simulink model "dsp_blr_AveOnly"  (R2018a)
settings: Solver=VariableStepAuto  StartTime=0.0  StopTime=100e-6  RelTol=1e-3
libraries: xrbsSSR_Library x26, xbsIndex_r4 x16, dspsigattribs x1, hdlsllib x1, simulink x1
(part 2 of 2)

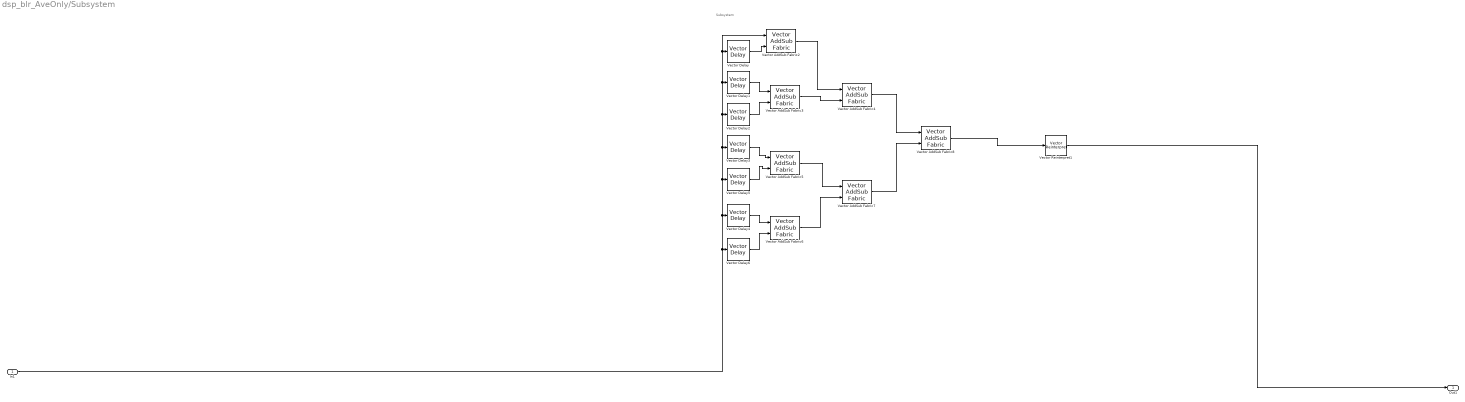
== system dsp_blr_AveOnly/Subsystem ==
  note: Subsystem
  In1 : Inport
  Vector AddSub Fabric{2..8} (7 alike) : xrbsSSR_Library/Vector AddSub Fabric  mode=Addition  use_carryin=off  use_carryout=off  en=off  sg_latency=0  precision=Full  arith_type=Unsigned  n_bits=16  bin_pt=14  quantization=Truncate  overflow=Wrap  use_behavioral_HDL=off  hw_selection=Fabric  pipelined=off  dbl_ovrd=off  block_type=addsub_ssr  sg_ssr=8  sg_ssr_prev=8  sg_ssr_name=vect_addsubfab
      settings: SourceProductName=Xilinx SSR Blockset
  Vector Delay : xrbsSSR_Library/Vector Delay  sg_latency=2  infoeditControl=Selection of Reset will increase slice count due to use of real FFs and instead of SRLs  en=off  vectorize_en=off  rst=off  reg_retiming=off  block_type=delay_ssr  dbl_ovrd=off  sg_ssr=8  sg_ssr_prev=8  sg_ssr_name=vect_delay
      settings: SourceProductName=Xilinx SSR Blockset
  Vector Delay1 : xrbsSSR_Library/Vector Delay  sg_latency=4  infoeditControl=Selection of Reset will increase slice count due to use of real FFs and instead of SRLs  en=off  vectorize_en=off  rst=off  reg_retiming=off  block_type=delay_ssr  dbl_ovrd=off  sg_ssr=8  sg_ssr_prev=8  sg_ssr_name=vect_delay
      settings: SourceProductName=Xilinx SSR Blockset
  Vector Delay2 : xrbsSSR_Library/Vector Delay  sg_latency=6  infoeditControl=Selection of Reset will increase slice count due to use of real FFs and instead of SRLs  en=off  vectorize_en=off  rst=off  reg_retiming=off  block_type=delay_ssr  dbl_ovrd=off  sg_ssr=8  sg_ssr_prev=8  sg_ssr_name=vect_delay
      settings: SourceProductName=Xilinx SSR Blockset
  Vector Delay3 : xrbsSSR_Library/Vector Delay  sg_latency=8  infoeditControl=Selection of Reset will increase slice count due to use of real FFs and instead of SRLs  en=off  vectorize_en=off  rst=off  reg_retiming=off  block_type=delay_ssr  dbl_ovrd=off  sg_ssr=8  sg_ssr_prev=8  sg_ssr_name=vect_delay
      settings: SourceProductName=Xilinx SSR Blockset
  Vector Delay4 : xrbsSSR_Library/Vector Delay  sg_latency=12  infoeditControl=Selection of Reset will increase slice count due to use of real FFs and instead of SRLs  en=off  vectorize_en=off  rst=off  reg_retiming=off  block_type=delay_ssr  dbl_ovrd=off  sg_ssr=8  sg_ssr_prev=8  sg_ssr_name=vect_delay
      settings: SourceProductName=Xilinx SSR Blockset
  Vector Delay5 : xrbsSSR_Library/Vector Delay  sg_latency=10  infoeditControl=Selection of Reset will increase slice count due to use of real FFs and instead of SRLs  en=off  vectorize_en=off  rst=off  reg_retiming=off  block_type=delay_ssr  dbl_ovrd=off  sg_ssr=8  sg_ssr_prev=8  sg_ssr_name=vect_delay
      settings: SourceProductName=Xilinx SSR Blockset
  Vector Delay6 : xrbsSSR_Library/Vector Delay  sg_latency=14  infoeditControl=Selection of Reset will increase slice count due to use of real FFs and instead of SRLs  en=off  vectorize_en=off  rst=off  reg_retiming=off  block_type=delay_ssr  dbl_ovrd=off  sg_ssr=8  sg_ssr_prev=8  sg_ssr_name=vect_delay
      settings: SourceProductName=Xilinx SSR Blockset
  Vector Reinterpret1 : xrbsSSR_Library/Vector Reinterpret  sg_ssr=8  sg_ssr_prev=8  force_arith_type=off  arith_type=Unsigned  force_bin_pt=on  bin_pt=7  block_type=reinterpret_ssr
      settings: SourceProductName=Xilinx SSR Blockset  infoedit="The Vector Reinterpret block Changes vector input signal type without altering the binary representation. You can change the signal between signed and unsigned, and relocate the binary point.<br><br>Hardware notes: In hardware this block costs nothing.<br><br>Example:  Suppose the input is 6 bits wide, signed, with 2 fractional bits, and the output is forced to unsigned with 0 fractional bits.  Then an input of -2.0 (1110.00 in binary 2's complement) becomes an output of 56 (111000 in binary)."
  Out1 : Outport
  wires:
  Vector AddSub Fabric6/1 -> Vector AddSub Fabric7/2
  In1/1 -> Vector AddSub Fabric2/1, Vector Delay/1, Vector Delay1/1, Vector Delay2/1, Vector Delay3/1, Vector Delay5/1, Vector Delay4/1, Vector Delay6/1
  Vector Delay3/1 -> Vector AddSub Fabric5/1
  Vector Delay/1 -> Vector AddSub Fabric2/2
  Vector AddSub Fabric2/1 -> Vector AddSub Fabric4/1
  Vector Delay2/1 -> Vector AddSub Fabric3/2
  Vector Delay6/1 -> Vector AddSub Fabric6/2
  Vector AddSub Fabric8/1 -> Vector Reinterpret1/1
  Vector Delay5/1 -> Vector AddSub Fabric5/2
  Vector AddSub Fabric3/1 -> Vector AddSub Fabric4/2
  Vector Delay4/1 -> Vector AddSub Fabric6/1
  Vector AddSub Fabric4/1 -> Vector AddSub Fabric8/1
  Vector AddSub Fabric7/1 -> Vector AddSub Fabric8/2
  Vector Delay1/1 -> Vector AddSub Fabric3/1
  Vector AddSub Fabric5/1 -> Vector AddSub Fabric7/1
  Vector Reinterpret1/1 -> Out1/1

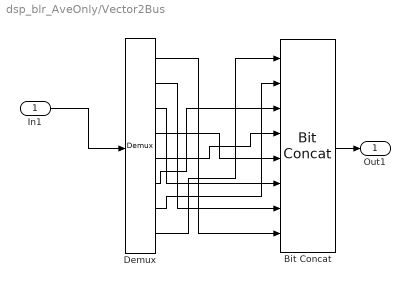
== system dsp_blr_AveOnly/Vector2Bus ==
  In1 : Inport
  Bit Concat : hdlsllib/Logic and Bit Operations/Bit Concat  numInputs=8
      settings: SourceProductName=HDL Coder  SourceProductBaseCode=HD
  Demux : Demux  Outputs=8
  Out1 : Outport
  wires:
  Demux/1 -> Bit Concat/8
  Demux/8 -> Bit Concat/1
  Demux/3 -> Bit Concat/6
  Bit Concat/1 -> Out1/1
  Demux/7 -> Bit Concat/2
  Demux/4 -> Bit Concat/5
  Demux/2 -> Bit Concat/7
  Demux/6 -> Bit Concat/3
  Demux/5 -> Bit Concat/4
  In1/1 -> Demux/1
